simulink model "EV314_test"  (Simulink 7.6)
settings: Solver=FixedStepDiscrete  StartTime=0.0  StopTime=Inf  RelTol=1e-3
libraries: simulink x4, rpi_blkst x1
settings Model: Creator=jacques  LastModifiedBy=jacques  SimulationMode=external
settings OptimizationCC: OptimizeModelRefInitCode=on  LifeSpan=1
settings HardwareCC: ProdIntDivRoundTo=Zero  ProdEndianess=LittleEndian  ProdHWDeviceType=Intel->x86/Pentium
settings RTWCC: SystemTargetFile=ert_rpi.tlc  TemplateMakefile=ert_rpi.tmf  PostCodeGenCommand=postGenFunc(buildInfo)  Description=RTW Embedded Coder RPI target  ProcessScript=ert_rpi_make_rtw_hook
settings CodeAppCC: IgnoreCustomStorageClasses=off
settings STFCustomTargetCC: ModelReferenceCompliant=off  CombineOutputUpdateFcns=on  ERTCustomFileBanners=on  SupportNonInlinedSFcns=off  SystemTargetFile=ert_rpi.tlc
settings ERTTargetCC: MultiwordLength=2048  ModelReferenceCompliant=off  ParMdlRefBuildCompliant=off  CompOptLevelCompliant=off  ERTFirstTimeCompliant=off  SupportContinuousTime=on  ModelStepFunctionPrototypeControlCompliant=off  CPPClassGenCompliant=off  ExtMode=on  ExtModeMexArgs='130.79.73.41'  InlinedParameterPlacement=NonHierarchical  ERTCustomFileTemplate=ert_rpi_file_process.tlc  ConvertIfToSwitch=off

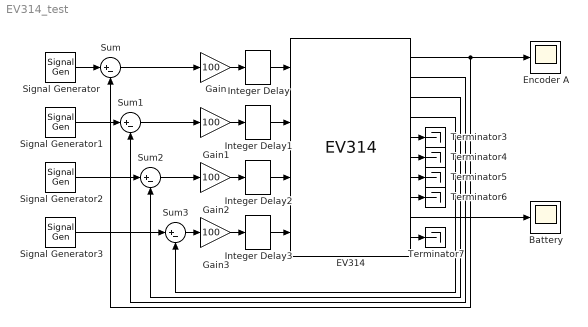
== system EV314_test ==
  Battery : Scope
      settings: YMin=0  YMax=2500
  EV314 : rpi_blkst/EV314  SystemSampleTime=-1  rpi_mask_ID=0  rpi_mask_Ts=0.01
  Encoder A : Scope
      settings: YMin=0  YMax=17.5
  Gain{,1..3} (4 alike) : Gain  Gain=100
  Integer Delay{,1..3} (4 alike) : simulink/Discrete/Integer Delay  NumDelays=1  vinit=0.0  samptime=-1
  Signal Generator{,1..3} (4 alike) : SignalGenerator  WaveForm=square  Amplitude=720  Frequency=0.25
  Sum{,1..3} (4 alike) : Sum  Inputs=|+-
  Terminator{3..7} (5 alike) : Terminator
  wires:
  EV314/1 -> Encoder A/1, Sum/2
  EV314/2 -> Sum1/2
  EV314/3 -> Sum2/2
  EV314/4 -> Sum3/2
  EV314/5 -> Terminator3/1
  EV314/6 -> Terminator4/1
  EV314/7 -> Terminator5/1
  EV314/8 -> Terminator6/1
  EV314/10 -> Terminator7/1
  EV314/9 -> Battery/1
  Signal Generator/1 -> Sum/1
  Sum/1 -> Gain/1
  Gain/1 -> Integer Delay/1
  Integer Delay/1 -> EV314/1
  Gain1/1 -> Integer Delay1/1
  Integer Delay1/1 -> EV314/2
  Gain2/1 -> Integer Delay2/1
  Gain3/1 -> Integer Delay3/1
  Integer Delay2/1 -> EV314/3
  Integer Delay3/1 -> EV314/4
  Sum1/1 -> Gain1/1
  Sum2/1 -> Gain2/1
  Sum3/1 -> Gain3/1
  Signal Generator1/1 -> Sum1/1
  Signal Generator2/1 -> Sum2/1
  Signal Generator3/1 -> Sum3/1
